simulink model "power_ForwardConverter_edit"  (R2018a)
settings: Solver=VariableStepAuto  StartTime=0.0  StopTime=0.02  MaxStep=1e-6  MinStep=1e-8  RelTol=1e-4  EnableMultiTasking=on
libraries: powerlib x18, simulink x1
Description:
  | Copyright 2008-2018 The MathWorks, Inc.
settings Model: Creator=MathWorks  LastModifiedBy=rmkna
settings SolverCC: ZeroCrossAlgorithm=Adaptive  SolverResetMethod=Robust
settings DataIOCC: ReturnWorkspaceOutputs=on
settings OptimizationCC: LifeSpan=inf
settings DebuggingCC: ReadBeforeWriteMsg=DisableAll  WriteAfterWriteMsg=DisableAll  WriteAfterReadMsg=DisableAll  IgnoredZcDiagnostic=none  MultiTaskDSMMsg=none  SFUnexpectedBacktrackingDiag=warning  SFNoUnconditionalDefaultTransitionDiag=warning  SFExecutionAtInitializationDiag=none
settings ModelReferenceCC: UpdateModelReferenceTargets=IfOutOfDate
settings SFSimCC: SFSimEcho=off
settings CodeAppCC: StateflowObjectComments=on
settings GRTTargetCC: TargetLangStandard=C89/C90 (ANSI)
settings ConfigComp: CovMetricSettings=dw  CovSaveCumulativeToWorkspaceVar=on  CovSaveSingleToWorkspaceVar=on  CovExternalEMLEnable=off
settings SimscapeCC: SimscapeNormalizeSystem=off  SimscapeNominalValues={1, 'bar'; 1, 'cm^3/s'; 1, 'bar*kg/s'; 1, 'kJ/kg'; 1, 'kW'; }

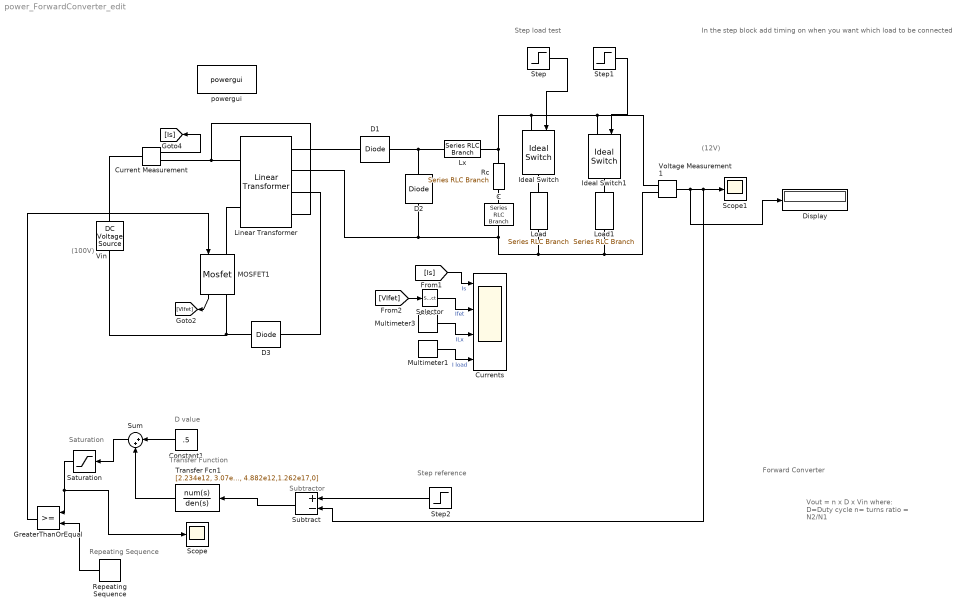
== system power_ForwardConverter_edit ==
  note: D value
  note: Repeating Sequence
  note: Step reference
  note: Subtractor
  note: Saturation
  note: Transfer Function
  note: In the step block add timing on when you want which load to be connected
  note: Step load test
  note: (12V)
  note: Vout = n x D x Vin
      | where: D=Duty cycle
      | n= turns ratio = N2/N1
  note: (100V)
  note: Forward Converter
  C : powerlib/Elements/Series RLC Branch  LConnTagsString=__new0  RConnTagsString=__new0  BranchType=C  Resistance=1e-4  Inductance=200e-6  SetiL0=off  InitialCurrent=0  Capacitance=100e-6  Setx0=off  InitialVoltage=0  Measurements=None
  Constant1 : Constant  Value=.5
  Current Measurement : powerlib/Measurements/Current Measurement  PhasorSimulation=off  OutputType=Complex  PSBequivalent=0
  Currents : Scope  NumInputPorts=4
  D1 : powerlib/Power Electronics/Diode  Ron=1e-3  Lon=0  Vf=0.8  IC=0  UseSnubber=off  Rs=inf  Cs=0  Measurements=off
  D2 : powerlib/Power Electronics/Diode  Ron=1e-3  Lon=0  Vf=0.7  IC=0  UseSnubber=off  Rs=inf  Cs=0  Measurements=off
  D3 : powerlib/Power Electronics/Diode  Ron=1e-3  Lon=0  Vf=0.8  IC=0  UseSnubber=off  Rs=inf  Cs=0  Measurements=off
  Display : Display
  GreaterThanOrEqual : RelationalOperator  OutDataTypeStr=boolean  RndMeth=Simplest
  Ideal Switch : powerlib/Power Electronics/Ideal Switch  Ron=0  Lon=0  IC=0  Rs=inf  Cs=inf  Measurements=off
  Ideal Switch1 : powerlib/Power Electronics/Ideal Switch  Ron=0  Lon=0  IC=0  Rs=inf  Cs=inf  Measurements=off
  Linear Transformer : powerlib/Elements/Linear Transformer  UNITS=SI  NominalPower=[ 75 100e3 ]  winding1=[100 0 0]  winding2=[24 0 0]  ThreeWindings=on  winding3=[100 0 0]  RmLm=[inf 10e-3]  Measurements=Magnetization current  DataType=on
  Load : powerlib/Elements/Series RLC Branch  LConnTagsString=__new0  RConnTagsString=__new0  BranchType=R  Resistance=5.6  Inductance=200e-6  SetiL0=off  InitialCurrent=0  Capacitance=400e-6  Setx0=off  InitialVoltage=0  Measurements=Branch current
  Load1 : powerlib/Elements/Series RLC Branch  LConnTagsString=__new0  RConnTagsString=__new0  BranchType=R  Resistance=5.6  Inductance=200e-6  SetiL0=off  InitialCurrent=0  Capacitance=400e-6  Setx0=off  InitialVoltage=0  Measurements=Branch current
  Lx : powerlib/Elements/Series RLC Branch  LConnTagsString=__new0  RConnTagsString=__new0  BranchType=L  Resistance=10  Inductance=50e-6  SetiL0=off  InitialCurrent=0  Capacitance=400e-6  Setx0=off  InitialVoltage=0  Measurements=Branch current
  MOSFET1 : powerlib/Power Electronics/Mosfet  Ron=1e-3  Lon=0  Rd=1e-3  Vfd=0  IC=0  Rs=1e6  Cs=inf  Measurements=on
  Multimeter1 : powerlib/Measurements/Multimeter  PhasorSimulation=off  OutputType=Complex  sel=1  L=7  Gain=1  yselected={'Ib: Load'};  PSBOutputType=1  PSBequivalent=0  AxesSetting=[0,0.1,-100,100]  Display=0  SavedBlockNames=-11
  Multimeter3 : powerlib/Measurements/Multimeter  PhasorSimulation=off  OutputType=Complex  sel=3  L=7  Gain=1  yselected={'Ib: Lx'};  PSBOutputType=1  PSBequivalent=0  AxesSetting=[0,0.1,-100,100]  Display=0  SavedBlockNames=-11
  Rc : powerlib/Elements/Series RLC Branch  LConnTagsString=__new0  RConnTagsString=__new0  BranchType=R  Resistance=50e-3  Inductance=200e-6  SetiL0=off  InitialCurrent=0  Capacitance=400e-6  Setx0=off  InitialVoltage=0  Measurements=Branch current
  Repeating Sequence : simulink/Sources/Repeating Sequence  rep_seq_t=[0 1/100e3]  rep_seq_y=[0 1]
  Saturation : Saturate  UpperLimit=0.8  LowerLimit=0.1
  Scope : Scope
  Scope1 : Scope
  Selector : Selector  InputPortWidth=2  IndexOptions=Index vector (dialog)  Indices=1  OutputSizes=1
  Step : Step  Time=0.001  Before=1  SampleTime=0
  Step1 : Step  Time=0.006  Before=1  After=0  SampleTime=0
  Step2 : Step  Time=0.008  Before=9.6  After=12  SampleTime=0
  Subtract : Sum  Inputs=+-
  Sum : Sum  Inputs=|++
  Transfer Fcn1 : TransferFcn  Numerator=[2.234e12, 3.07e16, 1.055e20]  Denominator=[4.72e7, 4.882e12,1.262e17,0]
  Vin : powerlib/Electrical Sources/DC Voltage Source  Amplitude=100  Measurements=None
  Voltage Measurement1 : powerlib/Measurements/Voltage Measurement  PhasorSimulation=off  OutputType=Complex  PSBequivalent=0
  powergui : powerlib/powergui  Priority=1  SimulationMode=Continuous  SampleTime=50e-6  frequency=60  Iterations=50  frequencyindice=0  Pbase=100e6  ErrMax=1e-4  UnitsV=kV  UnitsW=MW  buscounter=0  FunctionMessages=off  echomessages=off  EnableUseOfTLC=off  CurrentSourceSwitches=off  DisableSnubberDevices=off  DisableRonSwitches=off  DisableVfSwitches=off  DisplayEquations=off  SolverType=Tustin/Backward Euler (TBE)  Interpol=off  ExternalGateDelay=off  methode=off  Ts=100  x0status=blocks  SPID=on  SwTol=0  HookPort=off  RestoreLinks=warning  ResistiveCurrentMeasurement=off  Frange=[0:2:500]  Ylog=off  Xlog=on  ShowGrid=off  save=off  variable=ZData  structure=0  ZoomFFT=off  StartTime=0.0  cycles=1  DisplayStyle=1  fundamental=60  FreqAxis=off  MaxFrequency=1000  frequencyindicesteady=1  RmsSteady=1  display=off
  wires:
  MOSFET1/1 -> [VIfet]
  [VIfet] -> Selector/1
  Current Measurement/1 -> [Is]
  [Is] -> Currents/1  "Is"
  Multimeter3/1 -> Currents/3  "ILx"
  Selector/1 -> Currents/2  "Ifet"
  Voltage Measurement1/1 -> Display/1, Subtract/2, Scope1/1
  Repeating Sequence/1 -> GreaterThanOrEqual/2
  Multimeter1/1 -> Currents/4  "I load"
  Step1/1 -> Ideal Switch1/1
  Step/1 -> Ideal Switch/1
  Constant1/1 -> Sum/1
  Sum/1 -> Saturation/1
  Transfer Fcn1/1 -> Sum/2
  GreaterThanOrEqual/1 -> MOSFET1/1
  Saturation/1 -> Scope/1, GreaterThanOrEqual/1
  Step2/1 -> Subtract/1
  Subtract/1 -> Transfer Fcn1/1
  connections:
  Rc/LConn1 -- Lx/RConn1 -- Ideal Switch/LConn1 -- Ideal Switch1/LConn1 -- Voltage Measurement1/LConn1
  D2/LConn1 -- Load1/RConn1 -- Voltage Measurement1/LConn2 -- Load/RConn1 -- C/RConn1 -- Linear Transformer/RConn2
  Linear Transformer/LConn2 -- MOSFET1/LConn1
  Vin/LConn1 -- D3/LConn1 -- MOSFET1/RConn1
  Linear Transformer/RConn4 -- Current Measurement/RConn1 -- Linear Transformer/LConn1
  D1/LConn1 -- Linear Transformer/RConn1
  D2/RConn1 -- D1/RConn1 -- Lx/LConn1
  D3/RConn1 -- Linear Transformer/RConn3
  Vin/RConn1 -- Current Measurement/LConn1
  C/LConn1 -- Rc/RConn1
  Ideal Switch/RConn1 -- Load/LConn1
  Ideal Switch1/RConn1 -- Load1/LConn1
